simulink model "mavsim"  (R2020a)
settings: Solver=ode45  StartTime=0.0  StopTime=500  RelTol=1e-3  EnableMultiTasking=on
PreLoadFcn:
  | kalman_covariances
InitFcn:
  | param_quad
model workspace (MAT data in the model file):
  traj_x = [0 0.201 0.4 0.601 0.8 1 1.2 1.4 1.6 1.801 2 2.2 ... (4684 elements, 2342x2)]
  traj_y = [0 0.201 0.4 0.601 0.8 1 1.2 1.4 1.6 1.801 2 2.2 ... (4684 elements, 2342x2)]
  traj_z = [0 0.201 0.4 0.601 0.8 1 1.2 1.4 1.6 1.801 2 2.2 ... (4684 elements, 2342x2)]
  vel_x = [0 0 0.201 0.4 0.601 0.8 1 1.2 1.4 1.6 1.801 2 ... (4686 elements, 2343x2)]
  vel_y = [0 0 0.201 0.4 0.601 0.8 1 1.2 1.4 1.6 1.801 2 ... (4686 elements, 2343x2)]
  vel_z = [0 0 0.201 0.4 0.601 0.8 1 1.2 1.4 1.6 1.801 2 ... (4686 elements, 2343x2)]
undefined symbols (not defined in the file or in its folder): airdata, drawAircraft, P, plotmavstatevariables
libraries: simulink x5, sharedTrackingLibrary x1
(part 1 of 2)
settings Model: OrderedModelArguments=off  Creator=beard  LastModifiedBy=nsipes
settings DataIOCC: LimitDataPoints=on  SaveFormat=Array  ReturnWorkspaceOutputs=off
settings OptimizationCC: ExpressionDepthLimit=2147483647  InitFltsAndDblsToZero=on  LifeSpan=inf
settings DebuggingCC: UnderspecifiedInitializationDetection=Classic  MergeDetectMultiDrivingBlocksExec=none  SolverPrmCheckMsg=warning  MultiTaskDSMMsg=warning  MultiTaskCondExecSysMsg=none  StateNameClashWarn=warning  SFUnexpectedBacktrackingDiag=warning  SFNoUnconditionalDefaultTransitionDiag=warning  SFExecutionAtInitializationDiag=none  ArithmeticOperatorsInVariantConditions=warning
settings HardwareCC: ProdBitPerPointer=32  ProdBitPerSizeT=32  ProdBitPerPtrDiffT=32  ProdLargestAtomicFloat=None  ProdIntDivRoundTo=Undefined  ProdEndianess=Unspecified  ProdWordSize=32  ProdHWDeviceType=32-bit Generic
settings ModelReferenceCC: PropagateSignalLabelsOutOfModel=off
settings SFSimCC: SimUseLocalCustomCode=off  CustomCodeUndefinedFunction=UseInterfaceOnly
settings RTWCC: RTWUseLocalCustomCode=off
settings CodeAppCC: StateflowObjectComments=on
settings GRTTargetCC: TargetLangStandard=C89/C90 (ANSI)  CombineOutputUpdateFcns=off  GRTInterface=on
settings ConfigComp: CovMetricSettings=dw  CovHtmlReporting=on  CovSaveCumulativeToWorkspaceVar=on  CovSaveSingleToWorkspaceVar=on  CovExternalEMLEnable=off  CovSFcnEnable=off

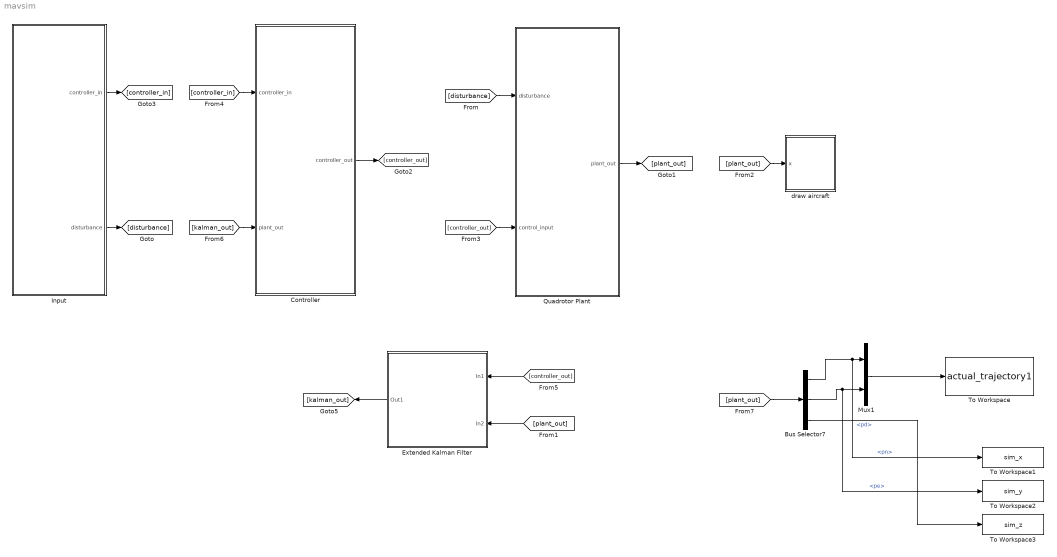
== system mavsim ==
  Bus Selector7 : BusSelector  OutputSignals=pn,pe,pd
  Controller : Subsystem
  Extended Kalman Filter : Subsystem
  Input : Subsystem
  Mux1 : Mux  Inputs=2
  Quadrotor Plant : Subsystem
  To Workspace : ToWorkspace  VariableName=actual_trajectory1  SaveFormat=Timeseries  SampleTime=-1
  To Workspace1 : ToWorkspace  VariableName=sim_x  SampleTime=0.25
      settings: Save2DSignal=2-D array (concatenate along first dimension)
  To Workspace2 : ToWorkspace  VariableName=sim_y  SampleTime=0.25
  To Workspace3 : ToWorkspace  VariableName=sim_z  SampleTime=0.25
  draw aircraft : Subsystem
      mask Display: image('icon.jpg')
  wires:
  Quadrotor Plant/1(plant_out) -> [plant_out]
  Input/2(disturbance) -> [disturbance]
  [disturbance] -> Quadrotor Plant/1(disturbance)
  [plant_out] -> draw aircraft/1(x)
  Controller/1(controller_out) -> [controller_out]
  [controller_out] -> Quadrotor Plant/2(control_input)
  Input/1(controller_in) -> [controller_in]
  [controller_in] -> Controller/1(controller_in)
  [controller_out] -> Extended Kalman Filter/1(In1)
  [plant_out] -> Extended Kalman Filter/2(In2)
  Extended Kalman Filter/1(Out1) -> [kalman_out]
  [kalman_out] -> Controller/2(plant_out)
  Mux1/1 -> To Workspace/1
  Bus Selector7/1 -> To Workspace1/1, Mux1/1  "<pn>"
  Bus Selector7/2 -> To Workspace2/1, Mux1/2  "<pe>"
  [plant_out] -> Bus Selector7/1
  Bus Selector7/3 -> To Workspace3/1  "<pd>"
